simulink model "Ch3_Simulation"  (R2024b)
settings: Solver=FixedStepDiscrete  StartTime=0  StopTime=511  FixedStep=1/128  RelTol=1e-3
undefined symbols (not defined in the file): gray
libraries: deeplib x1, dspfeatures x1
settings Model: Creator=The MathWorks, Inc.  LastModifiedBy=resjoehr
settings SolverCC: AlgebraicLoopSolver=TrustRegion
settings OptimizationCC: DefaultParameterBehavior=Inlined  EnhancedBackFolding=on  PassReuseOutputArgsThreshold=0  ZeroExternalMemoryAtStartup=off  ZeroInternalMemoryAtStartup=off  InitFltsAndDblsToZero=on  MaxStackSize=64  OptimizeBlockOrder=speed  DifferentSizesBufferReuse=on  OptimizationCustomize=off
settings DebuggingCC: ParameterTunabilityLossMsg=error  UnconnectedInputMsg=warning  UnconnectedOutputMsg=warning  UnconnectedLineMsg=warning
settings HardwareCC: ProdBitPerLong=64  ProdLongLongMode=on  ProdHWDeviceType=Intel->x86-64 (Linux 64)
settings ModelReferenceCC: EnableRefExpFcnMdlSchedulingChecks=on
settings SFSimCC: SimTargetLang=C++  SimGPUErrorChecks=on
settings RTWCC: GenerateReport=on  LaunchReport=on  CodeExecutionProfiling=on  TargetLang=C++  GPUComputeCapability=3.5  DLArmComputeVersion=19.05
settings CodeAppCC: ForceParamTrailComments=on  OperatorAnnotations=on
settings GRTTargetCC: TargetLangStandard=C++03 (ISO)  MatFileLogging=off  CodeInterfacePackaging=C++ class

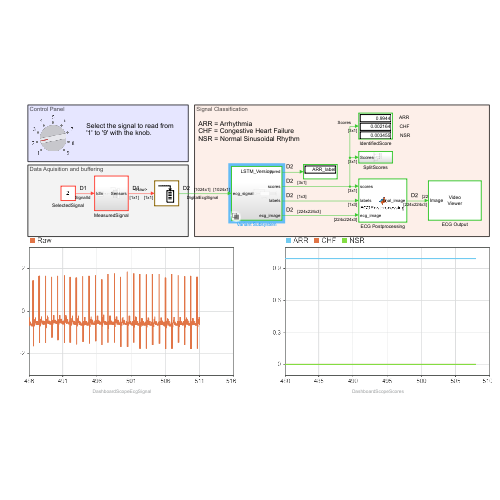
[thumbnail: Simulink's stored preview of the top-level diagram]
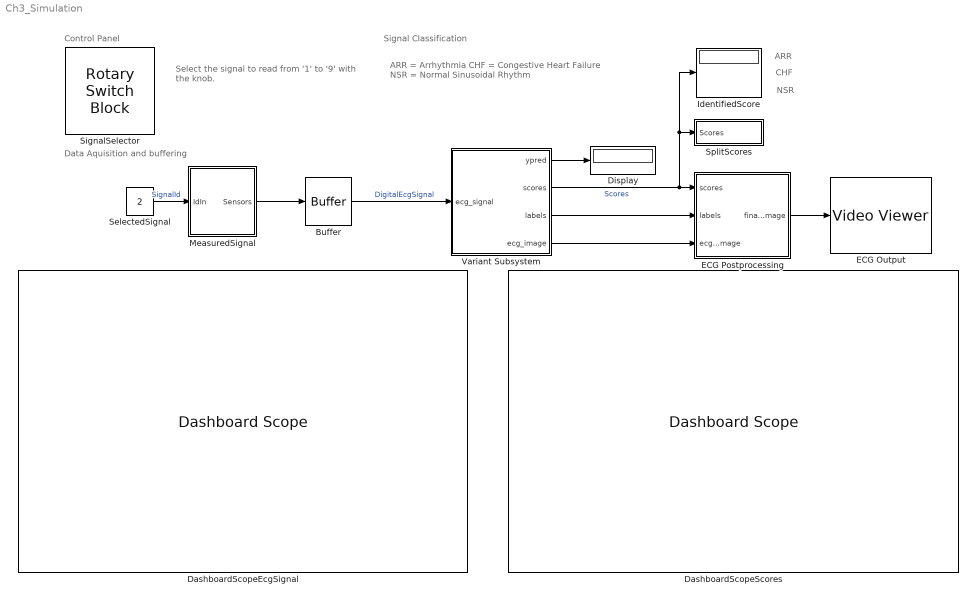
== system Ch3_Simulation ==
  note: ARR
  note: NSR
  note: ARR = Arrhythmia
      | CHF = Congestive Heart Failure
      | NSR = Normal Sinusoidal Rhythm
  note: Select the signal to read from '1' to '9' with the knob.
  note: Data Aquisition and buffering
  note: Control Panel
  note: CHF
  note: Signal Classification
  Buffer : Buffer  N=1024  V=512  OutputFrames=off
  DashboardScopeEcgSignal : DashboardScope  TimeSpan=30  ScaleAtStop=off  UpdateMode=Scroll
  DashboardScopeScores : DashboardScope  TimeSpan=30  Ymin=-0.1  Ymax=1.1  ScaleAtStop=off
  Display : Display
  ECG Output : VideoViewer  colormapValue=gray(256)  FigPos=[-1836.33333333333 840 592.666666666667 452]
  ECG Postprocessing : MATLAB Function  TreatAsAtomicUnit=on
  IdentifiedScore : Display
  MeasuredSignal : Subsystem  VariantControl=testMixed
  SelectedSignal : Constant  Value=2  SampleTime=-1
  SignalSelector : RotarySwitchBlock  LabelPosition=Hide
      settings: Values={{'1', '2', '3', '4', '5', '6', '7', '8', '9'}, [1 2 3 4 5 6 7 8 9]}
  SplitScores : Subsystem
  Variant Subsystem : Subsystem  Variant=on  VariantControlMode=label  LabelModeActiveChoice=true
  wires:
  ECG Postprocessing/1(final_image) -> ECG Output/1
  Variant Subsystem/3(labels) -> ECG Postprocessing/2(labels)
  Variant Subsystem/4(ecg_image) -> ECG Postprocessing/3(ecg_image)
  Variant Subsystem/1(ypred) -> Display/1
  Buffer/1 -> Variant Subsystem/1(ecg_signal)  "DigitalEcgSignal"
  Variant Subsystem/2(scores) -> ECG Postprocessing/1(scores), SplitScores/1(Scores), IdentifiedScore/1  "Scores"
  SelectedSignal/1 -> MeasuredSignal/1(IdIn)  "SignalId"
  MeasuredSignal/1(Sensors) -> Buffer/1

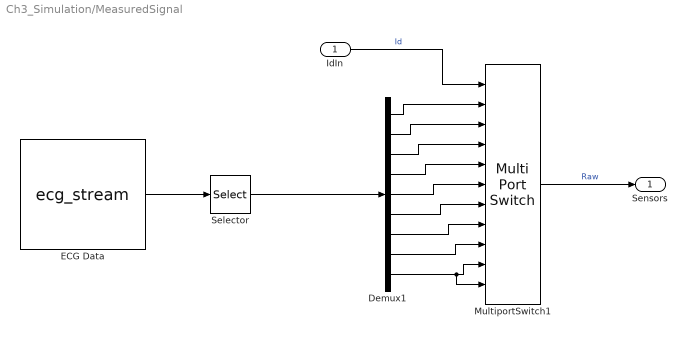
== system Ch3_Simulation/MeasuredSignal ==
  IdIn : Inport
  Demux1 : Demux  Outputs=9
  ECG Data : FromWorkspace  VariableName=ecg_stream  SampleTime=1/128
  MultiportSwitch1 : MultiPortSwitch  Inputs=9  DataPortForDefault=Additional data port  DiagnosticForDefault=None  SaturateOnIntegerOverflow=off  InputSameDT=off
  Selector : Selector  InputPortWidth=49  IndexOptions=Index vector (dialog)  Indices=[3 12 27 31 36 38 43 48 49]  OutputSizes=1
  Sensors : Outport
  wires:
  IdIn/1 -> MultiportSwitch1/1  "Id"
  Demux1/8 -> MultiportSwitch1/9
  Selector/1 -> Demux1/1
  Demux1/9 -> MultiportSwitch1/11, MultiportSwitch1/10
  Demux1/7 -> MultiportSwitch1/8
  Demux1/4 -> MultiportSwitch1/5
  Demux1/5 -> MultiportSwitch1/6
  MultiportSwitch1/1 -> Sensors/1  "Raw"
  ECG Data/1 -> Selector/1
  Demux1/6 -> MultiportSwitch1/7
  Demux1/1 -> MultiportSwitch1/2
  Demux1/3 -> MultiportSwitch1/4
  Demux1/2 -> MultiportSwitch1/3

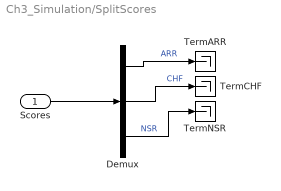
== system Ch3_Simulation/SplitScores ==
  Scores : Inport
  Demux : Demux  Outputs=3
  TermARR : Terminator
  TermCHF : Terminator
  TermNSR : Terminator
  wires:
  Scores/1 -> Demux/1
  Demux/2 -> TermCHF/1  "CHF"
  Demux/3 -> TermNSR/1  "NSR"
  Demux/1 -> TermARR/1  "ARR"

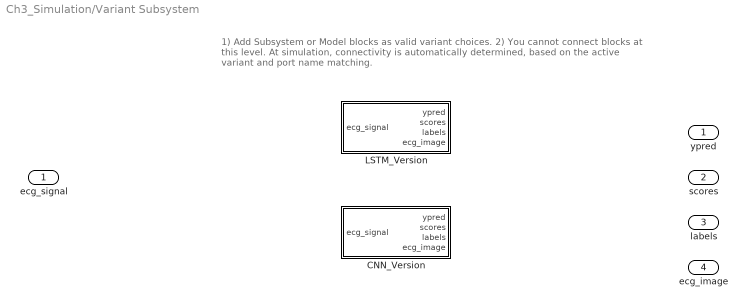
== system Ch3_Simulation/Variant Subsystem ==
  note: 1) Add Subsystem or Model blocks as valid variant choices.
      | 2) You cannot connect blocks at this level. At simulation, connectivity is automatically
      | determined, based on the active variant and port name matching.
  ecg_signal : Inport
  CNN_Version : Subsystem  VariantControl=false
  LSTM_Version : Subsystem  VariantControl=true
  ypred : Outport
  scores : Outport  Port=2
  labels : Outport  Port=3
  ecg_image : Outport  Port=4

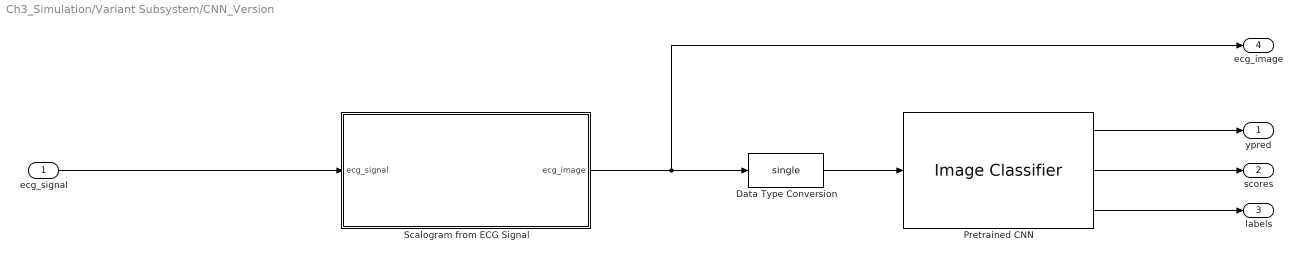
== system Ch3_Simulation/Variant Subsystem/CNN_Version ==
  ecg_signal : Inport
  Data Type Conversion : DataTypeConversion  OutDataTypeStr=single  SaturateOnIntegerOverflow=off  RndMeth=Floor
  "Pretrained CNN " : deeplib/Image Classifier  Network=Network from MAT-file  NetworkFunction=squeezenet  NetworkFilePath=trained_GN.mat  NetworkClassesVariable=classNames  MiniBatchSize=128  ResizeInput=on  Classification=on  Predictions=on  ForceInterpretedSim=off  PredictMode=All probabilities and labels  K=5
  Scalogram from ECG Signal : MATLAB Function  TreatAsAtomicUnit=on
  ypred : Outport
  scores : Outport  Port=2
  labels : Outport  Port=3
  ecg_image : Outport  Port=4
  wires:
  Data Type Conversion/1 -> "Pretrained CNN "/1
  Scalogram from ECG Signal/1(ecg_image) -> ecg_image/1, Data Type Conversion/1
  ecg_signal/1 -> Scalogram from ECG Signal/1(ecg_signal)
  "Pretrained CNN "/1 -> ypred/1
  "Pretrained CNN "/2 -> scores/1
  "Pretrained CNN "/3 -> labels/1

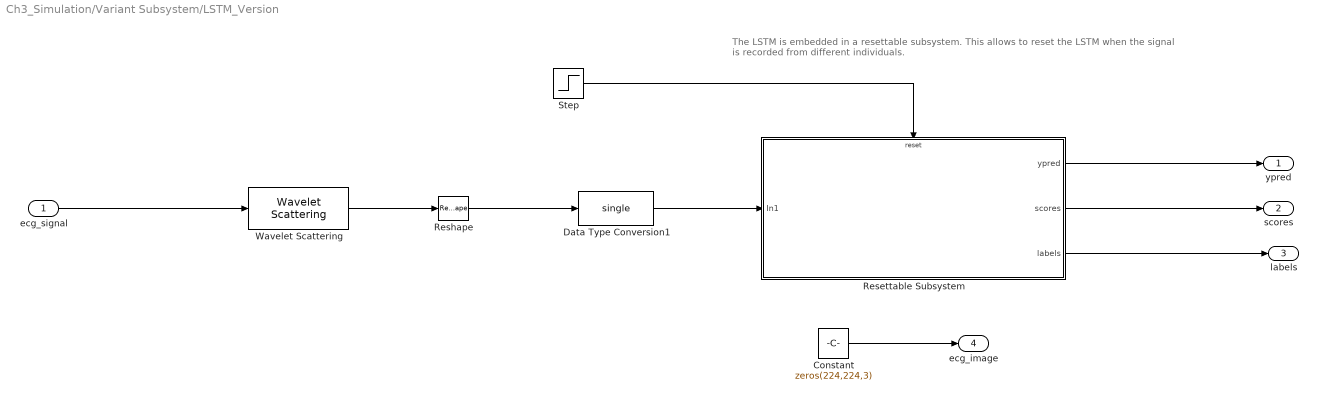
== system Ch3_Simulation/Variant Subsystem/LSTM_Version ==
  note: The LSTM is embedded in a resettable subsystem. This allows to reset the LSTM when the signal is recorded from different individuals.
  ecg_signal : Inport
  Constant : Constant  Value=zeros(224,224,3)  SampleTime=4
  Data Type Conversion1 : DataTypeConversion  OutDataTypeStr=single  SaturateOnIntegerOverflow=off  RndMeth=Floor
  Resettable Subsystem : Subsystem  TreatAsAtomicUnit=on
  Reshape : Reshape
  Step : Step  Time=0.1  SampleTime=4
  Wavelet Scattering : dspfeatures/Wavelet Scattering  SignalLength=1024  OverlapLength=0  SpecifySampleRate=on  SampleRate=128  InvarianceScaleSamples=512  InvarianceScaleSeconds=4  QualityFactors=[8,1]  OptimizePath=off  OversamplingFactor=0  Boundary=periodic  IncludeZeroOrderCoeff=on  FeatureMatrixNormalization=none  FeatureMatrixTransform=none
  ypred : Outport
  scores : Outport  Port=2
  labels : Outport  Port=3
  ecg_image : Outport  Port=4
  wires:
  Reshape/1 -> Data Type Conversion1/1
  ecg_signal/1 -> Wavelet Scattering/1
  Wavelet Scattering/1 -> Reshape/1
  Data Type Conversion1/1 -> Resettable Subsystem/1(In1)
  Constant/1 -> ecg_image/1
  Resettable Subsystem/2(scores) -> scores/1
  Resettable Subsystem/3(labels) -> labels/1
  Step/1 -> Resettable Subsystem/Reset
  Resettable Subsystem/1(ypred) -> ypred/1

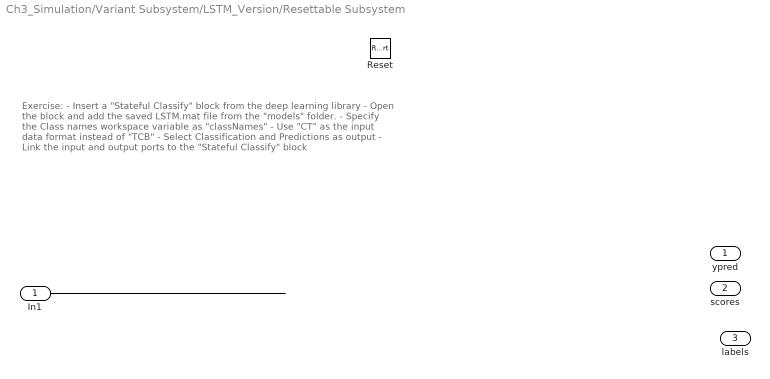
== system Ch3_Simulation/Variant Subsystem/LSTM_Version/Resettable Subsystem ==
  note: Exercise:
      | - Insert a "Stateful Classify" block from the deep learning library
      | - Open the block and add the saved LSTM.mat file from the "models" folder.
      | - Specify the Class names workspace variable as "classNames"
      | - Use "CT" as the input data format instead of "TCB"
      | - Select Classification and Predictions as output
      | - Link the input and output ports to the "Stateful Classify" block
  In1 : Inport
  Reset : ResetPort  DisableCoverage=on
  ypred : Outport
  scores : Outport  Port=2
  labels : Outport  Port=3
  wires:
  In1/1 -> ?
  ? -> ypred/1
  ? -> scores/1
  ? -> labels/1

== matlab function Ch3_Simulation/ECG Postprocessing ==
  data: scores input; labels input; ecg_image input; final_image output
function final_image = ECGPostprocessing(scores, labels, ecg_image)
    
    final_image = label_prob_image(ecg_image, scores, labels);

end

== matlab function Ch3_Simulation/Variant Subsystem/CNN_Version/Scalogram from ECG Signal ==
  data: ecg_signal input; ecg_image output
function ecg_image  = ScalogramFromECG(ecg_signal)
    
    ecg_image = ecg_to_scalogram(ecg_signal);  

end
